simulink model "uz_deadbeat_block"  (R2022a)
settings: Solver=FixedStepDiscrete  StartTime=0.0  StopTime=1  RelTol=1e-3
InitFcn:
  | clear all;
  | clc;
  | Ts = 25e-6;
libraries: spsCurrentMeasurementLib x3, spsSeriesRLCBranchLib x2, spsDCVoltageSourceLib x1, spsPWMGenerator2LevelLib x1, spsPermanentMagnetSynchronousMachineLib x1, spsTwoLevelConverterLib x1, spsabctodq0Lib x1, spspowerguiLib x1
settings Model: DataTypeOverride=Off  Creator=go98noz  LastModifiedBy=go98noz
settings SolverCC: AlgebraicLoopSolver=TrustRegion  AutoInsertRateTranBlk=on
settings DataIOCC: LimitDataPoints=on  SaveOutput=off  SaveTime=off
settings OptimizationCC: BlockReduction=off  ConditionallyExecuteInputs=off  DefaultParameterBehavior=Inlined  InheritOutputTypeSmallerThanSingle=on  LifeSpan=inf
settings DebuggingCC: AlgebraicLoopMsg=error  SingleTaskRateTransMsg=error  UnconnectedInputMsg=warning  UnconnectedOutputMsg=warning  UnconnectedLineMsg=warning  AllowSymbolicDim=off  StrictBusMsg=ErrorOnBusTreatedAsVector  SFUnexpectedBacktrackingDiag=warning  SFNoUnconditionalDefaultTransitionDiag=warning  SFExecutionAtInitializationDiag=none  SFMachineParentedDataDiag=warning  ArithmeticOperatorsInVariantConditions=warning
settings HardwareCC: ProdBitPerPointer=32  ProdBitPerSizeT=32  ProdBitPerPtrDiffT=32  ProdLargestAtomicFloat=None  ProdIntDivRoundTo=Undefined  ProdEndianess=Unspecified  ProdWordSize=32  ProdHWDeviceType=ASIC/FPGA->ASIC/FPGA  ProdEqTarget=off
settings SFSimCC: SimUseLocalCustomCode=off  CustomCodeUndefinedFunction=UseInterfaceOnly
settings RTWCC: RTWUseLocalCustomCode=off
settings CodeAppCC: StateflowObjectComments=on
settings GRTTargetCC: TargetLangStandard=C89/C90 (ANSI)
settings ConfigComp: CovScope=ReferencedModels  CovMetricSettings=dw  CovSaveCumulativeToWorkspaceVar=on  CovSaveSingleToWorkspaceVar=on  CovExternalEMLEnable=off  CovSFcnEnable=off

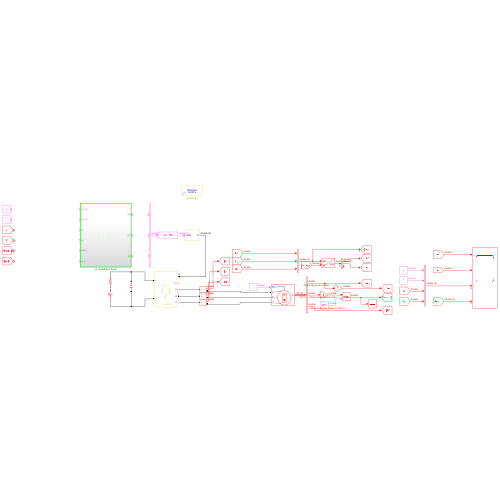
[thumbnail: Simulink's stored preview of the top-level diagram]
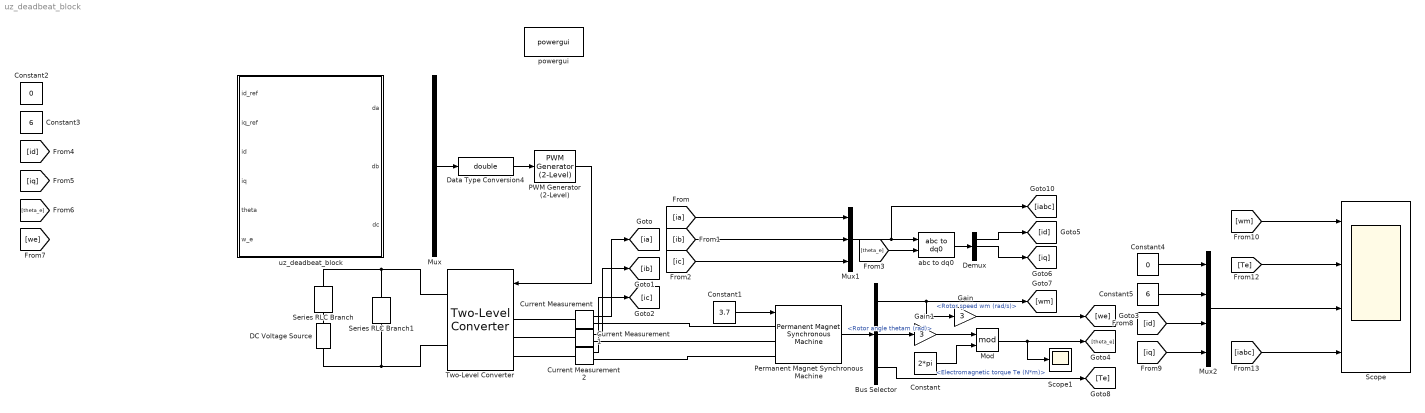
== system uz_deadbeat_block ==
  Bus Selector : BusSelector  OutputSignals=Rotor speed wm (rad/s),Rotor angle thetam (rad),Electromagnetic torque Te (N*m)
  Constant : Constant  Value=2*pi
  Constant1 : Constant  Value=3.7
  Constant2 : Constant  Value=0
  Constant3 : Constant  Value=6
  Constant4 : Constant  Value=0
  Constant5 : Constant  Value=6
  Current Measurement : spsCurrentMeasurementLib/Current Measurement  PhasorSimulation=off  OutputType=Complex  PSBequivalent=0
  Current Measurement1 : spsCurrentMeasurementLib/Current Measurement  PhasorSimulation=off  OutputType=Complex  PSBequivalent=0
  Current Measurement2 : spsCurrentMeasurementLib/Current Measurement  PhasorSimulation=off  OutputType=Complex  PSBequivalent=0
  DC Voltage Source : spsDCVoltageSourceLib/DC Voltage Source  Amplitude=340  Measurements=None
  Data Type Conversion4 : DataTypeConversion  OutDataTypeStr=double  SaturateOnIntegerOverflow=off  RndMeth=Floor
  Demux : Demux  Outputs=3
  Gain : Gain  Gain=3
  Gain1 : Gain  Gain=3
  Mod : Math  Operator=mod
  Mux : Mux  Inputs=3
  Mux1 : Mux  Inputs=3
  Mux2 : Mux
  PWM Generator (2-Level) : spsPWMGenerator2LevelLib/PWM Generator (2-Level)  ModulatorType=Three-phase bridge (6 pulses)  ModulatorMode=Unsynchronized  Fc=20e3  Pc=0  nF=27  MinMax="[ 0  1 ]"  SamplingTechnique=Asymmetrical regular (double edge)  ModulatingSignals=off  m=0.8  Freq=60  Phase=0  Ts=0  ShowCarrierOutport=off
  Permanent Magnet Synchronous Machine : spsPermanentMagnetSynchronousMachineLib/Permanent Magnet Synchronous Machine  NbPhases=3  FluxDistribution=Sinusoidal  RotorType=Round  MechanicalLoad=Torque Tm  PresetModel=No  ShowDetailedParameters=on  MeasurementBus=off  Resistance=1.2  Inductance=8.5e-3  dqInductances=[8.5e-3,8.5e-3]  La=0.0136  MachineConstant=Flux linkage established by magnets (V.s)  Flux=0.140  VoltageCst=76.1796  TorqueCst=0.63  Flat=120  Mechanical=[0.0002506 0.0004924 3 0]  PolePairs=4  InitialConditions=[100,0, 0,0]  InitialConditions5ph=[0 0 0 0 0 0]  RefAngle=Aligned with phase A axis (original Park)  IterativeDiscreteModel=Trapezoidal non iterative  TsBlock=-1  TsPowergui=0
  Scope : Scope  NumInputPorts=4
  Scope1 : Scope
  Series RLC Branch : spsSeriesRLCBranchLib/Series RLC Branch  LConnTagsString=__new0  RConnTagsString=__new0  BranchType=R  Resistance=1e-3  Inductance=1e-3  SetiL0=off  InitialCurrent=0  Capacitance=1e-6  Setx0=off  InitialVoltage=0  Measurements=None
  Series RLC Branch1 : spsSeriesRLCBranchLib/Series RLC Branch  LConnTagsString=__new0  RConnTagsString=__new0  BranchType=C  Resistance=1e-3  Inductance=1e-3  SetiL0=off  InitialCurrent=0  Capacitance=3300e-6  Setx0=off  InitialVoltage=0  Measurements=None
  Two-Level Converter : spsTwoLevelConverterLib/Two-Level Converter  ModelType=Switching devices  Ron=1e-3  Rs=1e6  Cs=inf  Vforward=[0,0]  Ron_Diode=1e-3  Rs_Diode=1e6  Cs_Diode=inf  Vf_Diode=1e-3  Rs_CurrentSource=inf  Ron_ACsource=1e-3
      settings: SourceProductBaseCode=PS
  abc to dq0 : spsabctodq0Lib/abc to dq0  Alignment=Aligned with phase A axis
  powergui : spspowerguiLib/powergui  Priority=1  SimulationMode=Discrete  SampleTime=1e-6  frequency=60  Iterations=50  frequencyindice=0  Pbase=100e6  ErrMax=1e-4  UnitsV=kV  UnitsW=MW  buscounter=0  FunctionMessages=off  echomessages=off  EnableUseOfTLC=off  CurrentSourceSwitches=off  DisableSnubberDevices=off  DisableRonSwitches=off  DisableVfSwitches=off  DisplayEquations=off  AutomaticDiscreteSolvers=off  SolverType=Tustin/Backward Euler (TBE)  Interpol=off  ExternalGateDelay=off  methode=off  Ts=100  x0status=blocks  SPID=on  SwTol=0  HookPort=off  NonlinearTolerance=1e-4  nMaxIteration=100  ContinueOnMaxIteration=off  RestoreLinks=warning  ResistiveCurrentMeasurement=off  Frange=[0:2:500]  Ylog=off  Xlog=on  ShowGrid=off  save=off  variable=ZData  structure=0  ZoomFFT=off  StartTime=0.0  cycles=1  DisplayStyle=1  fundamental=60  FreqAxis=off  MaxFrequency=1000  frequencyindicesteady=1  RmsSteady=1  display=off
  uz_deadbeat_block : Subsystem  TreatAsAtomicUnit=on
  wires:
  Current Measurement/1 -> [ia]
  Current Measurement1/1 -> [ib]
  Current Measurement2/1 -> [ic]
  Permanent Magnet Synchronous Machine/1 -> Bus Selector/1
  Bus Selector/1 -> Gain/1, [wm]  "<Rotor speed wm (rad/s)>"
  Bus Selector/2 -> Gain1/1  "<Rotor angle thetam (rad)>"
  Constant/1 -> Mod/2
  Gain1/1 -> Mod/1
  Constant1/1 -> Permanent Magnet Synchronous Machine/1
  Mux1/1 -> [iabc], abc to dq0/1
  [theta_e] -> abc to dq0/2
  abc to dq0/1 -> Demux/1
  Demux/1 -> [id]
  Demux/2 -> [iq]
  Constant4/1 -> Mux2/1
  Constant5/1 -> Mux2/2
  [id] -> Mux2/3
  [iq] -> Mux2/4
  [ia] -> Mux1/1
  [ib] -> Mux1/2
  [ic] -> Mux1/3
  Gain/1 -> [we]
  Mod/1 -> [theta_e], Scope1/1
  Data Type Conversion4/1 -> PWM Generator (2-Level)/1
  Bus Selector/3 -> [Te]  "<Electromagnetic torque Te (N*m)>"
  [wm] -> Scope/1
  [Te] -> Scope/2
  Mux2/1 -> Scope/3
  [iabc] -> Scope/4
  PWM Generator (2-Level)/1 -> Two-Level Converter/1
  Mux/1 -> Data Type Conversion4/1
  connections:
  Current Measurement/LConn1 -- Two-Level Converter/LConn1
  Current Measurement/RConn1 -- Permanent Magnet Synchronous Machine/LConn1
  Two-Level Converter/LConn2 -- Current Measurement1/LConn1
  Current Measurement1/RConn1 -- Permanent Magnet Synchronous Machine/LConn2
  Current Measurement2/LConn1 -- Two-Level Converter/LConn3
  Current Measurement2/RConn1 -- Permanent Magnet Synchronous Machine/LConn3
  Series RLC Branch/RConn1 -- DC Voltage Source/RConn1
  Series RLC Branch/LConn1 -- Two-Level Converter/RConn1 -- Series RLC Branch1/LConn1
  DC Voltage Source/LConn1 -- Series RLC Branch1/RConn1 -- Two-Level Converter/RConn2

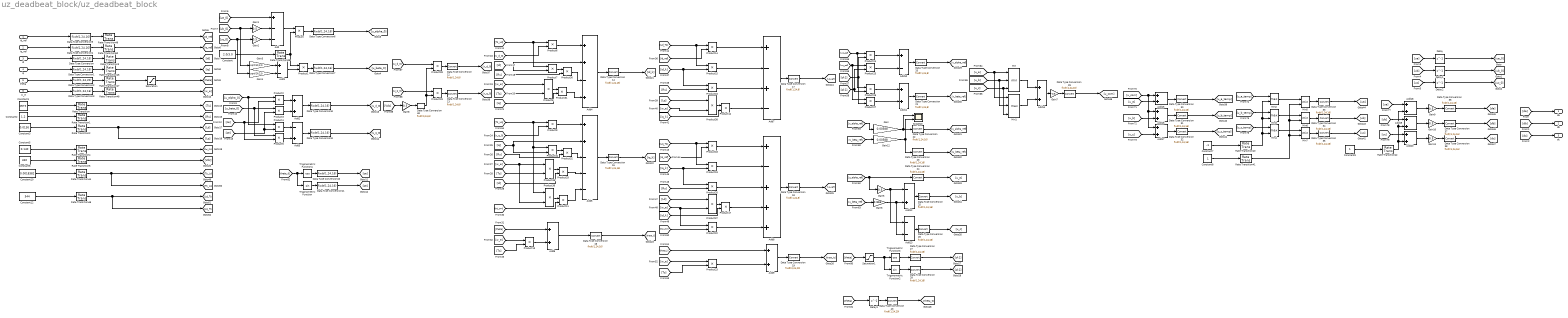
== system uz_deadbeat_block/uz_deadbeat_block ==
  id_ref : Inport
  iq_ref : Inport  Port=2
  id : Inport  Port=3
  iq : Inport  Port=4
  theta : Inport  Port=5
  w_e : Inport  Port=6
  Add : Sum  Inputs=+--
  Add1 : Sum  Inputs=+-
  Add10 : Sum  Inputs=+-
  Add{2,6,9,11,14..20} (11 alike) : Sum
  Add12 : Sum  Inputs=-+
  Add13 : Sum  Inputs=--
  Add3 : Sum  Inputs=-+
  Add4 : Sum  Inputs=++-+
  Add5 : Sum  Inputs=++---
  Add7 : Sum  Inputs=+-+-
  Add8 : Sum  Inputs=+-+++
  Constant : Constant  Value=2.0/3.0  OutDataTypeStr=fixdt(1,24,16)  SampleTime=-1
  Constant1 : Constant  Value=25e-6  OutDataTypeStr=fixdt(0,32,30)  SampleTime=-1
  Constant10 : Constant  Value=0.0018382  OutDataTypeStr=fixdt(0,24,22)  SampleTime=-1
  Constant12 : Constant  Value=544  OutDataTypeStr=fixdt(0,24,8)  SampleTime=-1
  Constant2 : Constant  Value=1.2  OutDataTypeStr=fixdt(1,24,18)  SampleTime=-1
  Constant3 : Constant  Value=0.0136  OutDataTypeStr=fixdt(0,24,20)  SampleTime=-1
  Constant5 : Constant  Value=0.140  OutDataTypeStr=fixdt(0,24,22)  SampleTime=-1
  Constant6 : Constant  Value=340  OutDataTypeStr=fixdt(0,24,8)  SampleTime=-1
  Constant7 : Constant  Value=-1  OutDataTypeStr=fixdt(1,24,16)  SampleTime=-1
  Constant8 : Constant  OutDataTypeStr=fixdt(1,24,16)  SampleTime=-1
  Constant9 : Constant  OutDataTypeStr=fixdt(1,24,16)  SampleTime=-1
  Data Type Conversion{,1,3..11,14..16,22..38} (31 alike) : DataTypeConversion  OutDataTypeStr=fixdt(1,24,16)  SaturateOnIntegerOverflow=off  RndMeth=Floor
  Data Type Conversion{12..13,17..18,20..21} (6 alike) : DataTypeConversion  OutDataTypeStr=fixdt(1,24,8)  SaturateOnIntegerOverflow=off  RndMeth=Floor
  Data Type Conversion19 : DataTypeConversion  OutDataTypeStr=fixdt(0,24,20)  SaturateOnIntegerOverflow=off  RndMeth=Floor
  Data Type Conversion2 : DataTypeConversion  OutDataTypeStr=fixdt(1,24,20)  SaturateOnIntegerOverflow=off  RndMeth=Floor
  Data Type Conversion43 : DataTypeConversion  OutDataTypeStr=fixdt(1,24,20)  SaturateOnIntegerOverflow=off  RndMeth=Floor
  Data Type Conversion48 : DataTypeConversion  OutDataTypeStr=fixdt(0,24,8)  SaturateOnIntegerOverflow=off  RndMeth=Floor
  Delay{,1..3} (4 alike) : Delay  DelayLength=1  InitialCondition=0  SampleTime=25e-6
  Gain : Gain  Gain=0.00588
  Gain{1..2,5,8..11} (7 alike) : Gain  Gain=0.5
  Gain12 : Gain  Gain=0.00588
  Gain3 : Gain  Gain=sqrt(3)/2.0
  Gain4 : Gain  Gain=sqrt(3)/2.0
  Gain6 : Gain  Gain=0.866
  Gain7 : Gain  Gain=-0.5
  Min : MinMax  Inputs=3
  Min1 : MinMax  Function=max  Inputs=3
  Min2 : MinMax  Function=max  Inputs=2
  Min3 : MinMax  Function=max  Inputs=2
  Min4 : MinMax  Function=max  Inputs=2
  Min5 : MinMax  Inputs=2
  Min6 : MinMax  Inputs=2
  Min7 : MinMax  Inputs=2
  Product{,1..9,11..20,22..38} (37 alike) : Product
  Rate Transition{,1..5,39..42,44..50} (17 alike) : RateTransition  OutPortSampleTime=25e-6
  Saturation : Saturate  UpperLimit=6.283  LowerLimit=0
  Saturation1 : Saturate  UpperLimit=6.283  LowerLimit=0
  Scope10 : Scope  NumInputPorts=2
  Trigonometric Function : Trigonometry  ApproximationMethod=CORDIC
  Trigonometric Function1 : Trigonometry  Operator=cos  ApproximationMethod=CORDIC
  Trigonometric Function2 : Trigonometry  ApproximationMethod=CORDIC
  Trigonometric Function3 : Trigonometry  Operator=cos  ApproximationMethod=CORDIC
  da : Outport  VectorParamsAs1DForOutWhenUnconnected=off
  db : Outport  Port=2  VectorParamsAs1DForOutWhenUnconnected=off
  dc : Outport  Port=3  VectorParamsAs1DForOutWhenUnconnected=off
  wires:
  [da] -> da/1
  [db] -> db/1
  [dc] -> dc/1
  [ua] -> Delay/1
  [ub] -> Delay1/1
  [uc] -> Delay2/1
  [ua_0] -> Add/1
  [ub_0] -> Gain3/1, Gain1/1
  [uc_0] -> Gain4/1, Gain2/1
  Gain1/1 -> Add/2
  Gain2/1 -> Add/3
  Add/1 -> Product/1
  Gain3/1 -> Add1/1
  Gain4/1 -> Add1/2
  Add1/1 -> Product1/2
  [theta_0] -> Trigonometric Function1/1, Trigonometric Function/1
  [u_alpha_0] -> Product4/1, Product2/1
  [ce] -> Product5/2, Product2/2
  [u_beta_0] -> Product5/1, Product3/1
  [se] -> Product3/2, Product4/2
  Product2/1 -> Add2/1
  Product3/1 -> Add2/2
  Product5/1 -> Add3/2
  Product4/1 -> Add3/1
  [Ts_Ld] -> Product7/1, Product6/1
  [v_d_0] -> Product6/2
  Product6/1 -> Add4/1
  [id] -> Product7/2, Add4/2
  [Rs] -> Product30/2
  [w_e] -> Product8/1
  [Ts] -> Product8/2
  Product33/1 -> Add5/4
  [id] -> Product33/2
  [Ts] -> Product35/2
  [w_e] -> Product36/2, Product35/1
  [Rs] -> Product32/2
  [iq] -> Product34/2, Add5/2
  Product9/1 -> Add5/1
  [v_q_0] -> Product9/2
  [Ts_Lq] -> Product9/1, Product36/1, Product34/1
  [Psi_PM] -> Product11/2
  Product11/1 -> Add5/5
  [w_e] -> Product13/1
  [Ts] -> Product13/2
  Product13/1 -> Add6/2
  [theta] -> Add6/1
  [Ld_Ts] -> Product15/1, Product14/1
  [id_ref] -> Product14/2
  Product14/1 -> Add7/1
  [id_k] -> Product16/1, Product15/2
  Product15/1 -> Add7/2
  [Rs] -> Product16/2
  Product16/1 -> Add7/3
  [Lq] -> Product38/1
  [w_e] -> Product38/2
  [iq_k] -> Product12/2
  Product12/1 -> Add7/4
  Product17/1 -> Add8/4
  [id_k] -> Product17/2
  [w_e] -> Product22/1, Product37/2
  [Ld] -> Product37/1
  Product20/1 -> Add8/3
  [Rs] -> Product20/2
  Product19/1 -> Add8/2
  [iq_k] -> Product19/2, Product20/1
  Product18/1 -> Add8/1
  [iq_ref] -> Product18/2
  [Lq_Ts] -> Product18/1, Product19/1
  [Psi_PM] -> Product22/2
  Product22/1 -> Add8/5
  [theta_k] -> Add9/1
  Product23/1 -> Add9/2
  [Ts] -> Product23/2
  [w_e] -> Product23/1
  [theta] -> Saturation1/1
  [vd_ref] -> Product26/1, Product24/1
  [ck1] -> Product24/2, Product27/2
  Product24/1 -> Add10/1
  [vq_ref] -> Product27/1, Product25/1
  [sk1] -> Product25/2, Product26/2
  Product25/1 -> Add10/2
  Product26/1 -> Add11/1
  Product27/1 -> Add11/2
  [v_alpha_ref] -> Gain/1
  [u_alpha_ref] -> Data Type Conversion24/1, Gain5/1
  Gain5/1 -> Add12/1, Add13/1
  [u_beta_ref] -> Gain6/1
  Gain6/1 -> Add12/2, Add13/2
  [u_b] -> Min1/2, Min/2
  [u_c] -> Min1/3, Min/3
  [u_a] -> Min1/1, Min/1
  Min/1 -> Add14/1
  Min1/1 -> Add14/2
  Add14/1 -> Gain7/1
  [u_d_0] -> Product28/1
  [Vdc] -> Gain8/1
  Gain8/1 -> Data Type Conversion48/1
  [u_q_0] -> Product29/1
  [u_com] -> Add17/1, Add16/1, Add15/1
  [u_a] -> Add15/2
  [u_b] -> Add16/2
  [u_c] -> Add17/2
  [u_a_temp] -> Min2/1
  [u_b_temp] -> Min3/1
  [u_c_temp] -> Min4/1
  Min2/1 -> Min5/1
  Min3/1 -> Min6/1
  Min4/1 -> Min7/1
  [ua] -> Add18/1
  [ub] -> Add19/1
  [uc] -> Add20/1
  Add18/1 -> Gain9/1
  Add19/1 -> Gain10/1
  Add20/1 -> Gain11/1
  Constant1/1 -> Rate Transition/1
  Rate Transition/1 -> [Ts]
  Constant2/1 -> Rate Transition1/1
  Constant3/1 -> Rate Transition2/1
  Constant6/1 -> Rate Transition5/1
  Constant5/1 -> Rate Transition4/1
  Rate Transition1/1 -> [Rs]
  Rate Transition2/1 -> [Lq], [Ld]
  Rate Transition4/1 -> [Psi_PM]
  Rate Transition5/1 -> [Vdc]
  Product/1 -> Data Type Conversion6/1
  Data Type Conversion6/1 -> [u_alpha_0]
  Product1/1 -> Data Type Conversion7/1
  Data Type Conversion7/1 -> [u_beta_0]
  Add2/1 -> Data Type Conversion8/1
  Data Type Conversion8/1 -> [u_d_0]
  Add3/1 -> Data Type Conversion9/1
  Data Type Conversion9/1 -> [u_q_0]
  Trigonometric Function1/1 -> Data Type Conversion10/1
  Data Type Conversion10/1 -> [ce]
  Trigonometric Function/1 -> Data Type Conversion11/1
  Data Type Conversion11/1 -> [se]
  Product28/1 -> Data Type Conversion12/1
  Data Type Conversion12/1 -> [v_d_0]
  Data Type Conversion13/1 -> [v_q_0]
  Product29/1 -> Data Type Conversion13/1
  Add4/1 -> Data Type Conversion14/1
  Data Type Conversion14/1 -> [id_k]
  Add5/1 -> Data Type Conversion15/1
  Data Type Conversion15/1 -> [iq_k]
  Add6/1 -> Data Type Conversion16/1
  Data Type Conversion16/1 -> [theta_k]
  Data Type Conversion17/1 -> [vd_ref]
  Add7/1 -> Data Type Conversion17/1
  Add8/1 -> Data Type Conversion18/1
  Data Type Conversion18/1 -> [vq_ref]
  Add9/1 -> Data Type Conversion19/1
  Data Type Conversion19/1 -> [theta_k1]
  Add10/1 -> Data Type Conversion20/1
  Data Type Conversion20/1 -> [v_alpha_ref]
  Add11/1 -> Data Type Conversion21/1
  Data Type Conversion21/1 -> [v_beta_ref]
  Gain/1 -> Scope10/1, Data Type Conversion22/1
  Data Type Conversion22/1 -> [u_alpha_ref]
  Gain12/1 -> Data Type Conversion23/1, Scope10/2
  Data Type Conversion23/1 -> [u_beta_ref]
  Data Type Conversion24/1 -> [u_a]
  Add12/1 -> Data Type Conversion25/1
  Data Type Conversion25/1 -> [u_b]
  Add13/1 -> Data Type Conversion26/1
  Data Type Conversion26/1 -> [u_c]
  Trigonometric Function3/1 -> Data Type Conversion27/1
  Data Type Conversion27/1 -> [ck1]
  Trigonometric Function2/1 -> Data Type Conversion28/1
  Data Type Conversion28/1 -> [sk1]
  Gain7/1 -> Data Type Conversion29/1
  Data Type Conversion29/1 -> [u_com]
  Add15/1 -> Data Type Conversion30/1
  Data Type Conversion30/1 -> [u_a_temp]
  Add16/1 -> Data Type Conversion31/1
  Data Type Conversion31/1 -> [u_b_temp]
  Add17/1 -> Data Type Conversion32/1
  Data Type Conversion32/1 -> [u_c_temp]
  Min5/1 -> Data Type Conversion33/1
  Data Type Conversion33/1 -> [ua]
  Min6/1 -> Data Type Conversion34/1
  Data Type Conversion34/1 -> [ub]
  Min7/1 -> Data Type Conversion35/1
  Data Type Conversion35/1 -> [uc]
  Gain9/1 -> Data Type Conversion36/1
  Data Type Conversion36/1 -> [da]
  Gain10/1 -> Data Type Conversion37/1
  Data Type Conversion37/1 -> [db]
  Gain11/1 -> Data Type Conversion38/1
  Data Type Conversion38/1 -> [dc]
  Constant/1 -> Rate Transition39/1
  Rate Transition39/1 -> Product/2, Product1/1
  Constant7/1 -> Rate Transition40/1
  Rate Transition40/1 -> Min4/2, Min3/2, Min2/2
  Constant8/1 -> Rate Transition41/1
  Rate Transition41/1 -> Min7/2, Min6/2, Min5/2
  Constant9/1 -> Rate Transition42/1
  Rate Transition42/1 -> Add20/2, Add19/2, Add18/2
  Delay/1 -> [ua_0]
  Delay1/1 -> [ub_0]
  Delay2/1 -> [uc_0]
  [v_beta_ref] -> Gain12/1
  Saturation/1 -> [theta]
  Saturation1/1 -> Trigonometric Function3/1, Trigonometric Function2/1
  [theta] -> Delay3/1
  Delay3/1 -> Data Type Conversion43/1
  Data Type Conversion43/1 -> [theta_0]
  Product7/1 -> Product30/1
  Product30/1 -> Add4/3
  Product8/1 -> Product31/1
  [iq] -> Product31/2
  Product31/1 -> Add4/4
  Product34/1 -> Product32/1
  Product35/1 -> Product33/1
  Product32/1 -> Add5/3
  Product36/1 -> Product11/1
  Product38/1 -> Product12/1
  Product37/1 -> Product17/1
  Rate Transition44/1 -> [Ts_Lq], [Ts_Ld]
  Rate Transition46/1 -> [Lq_Ts], [Ld_Ts]
  Constant12/1 -> Rate Transition46/1
  Data Type Conversion48/1 -> Product29/2, Product28/2
  Constant10/1 -> Rate Transition44/1
  Data Type Conversion3/1 -> Rate Transition48/1
  Data Type Conversion5/1 -> Rate Transition49/1
  Data Type Conversion/1 -> Rate Transition3/1
  Data Type Conversion1/1 -> Rate Transition45/1
  Data Type Conversion4/1 -> Rate Transition50/1
  Data Type Conversion2/1 -> Rate Transition47/1
  id_ref/1 -> Data Type Conversion5/1
  Rate Transition49/1 -> [id_ref]
  iq_ref/1 -> Data Type Conversion4/1
  Rate Transition50/1 -> [iq_ref]
  id/1 -> Data Type Conversion/1
  Rate Transition3/1 -> [id]
  iq/1 -> Data Type Conversion1/1
  Rate Transition45/1 -> [iq]
  theta/1 -> Data Type Conversion2/1
  Rate Transition47/1 -> Saturation/1
  w_e/1 -> Data Type Conversion3/1
  Rate Transition48/1 -> [w_e]
